simulink model "test"  (R2024b)
settings: Solver=VariableStepAuto  StartTime=0.0  StopTime=1  RelTol=1e-3
model workspace (MAT data in the model file):
  branch = 1
  resist = 1
values from neighbouring files (symbols this model uses):
  V = ww.ScopeData2.signals.values    [main.m]
libraries: spsCurrentMeasurementLib x1, spsPermanentMagnetSynchronousMachineLib x1, spsSeriesRLCBranchLib x1, spsUniversalBridgeLib x1, spsVoltageMeasurementLib x1, spsWindTurbineLib x1, sps_lib x1
settings Model: Creator=laity  LastModifiedBy=laity

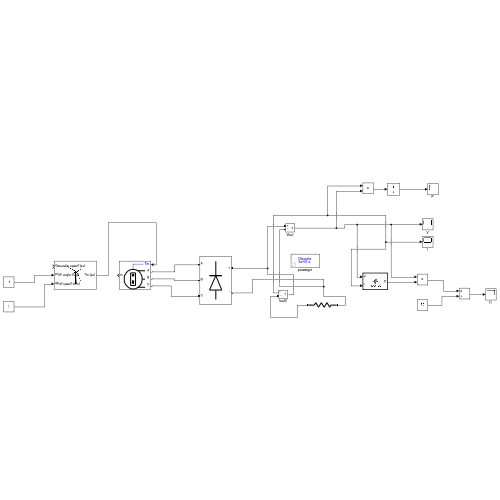
[thumbnail: Simulink's stored preview of the top-level diagram]
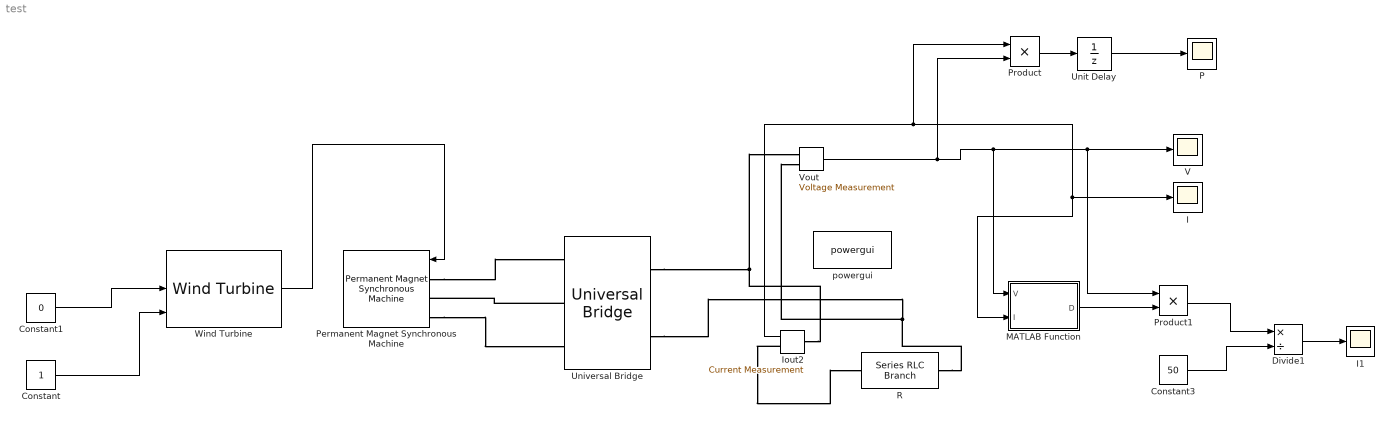
== system test ==
  Constant : Constant
  Constant1 : Constant  Value=0
  Constant3 : Constant  Value=50
  Divide1 : Product  Inputs=*/
  I : Scope
  I1 : Scope
  Iout2 : spsCurrentMeasurementLib/Current Measurement  PhasorSimulation=off  OutputType=Complex  PSBequivalent=0
  MATLAB Function : MATLAB Function  TreatAsAtomicUnit=on
  P : Scope
  Permanent Magnet Synchronous Machine : spsPermanentMagnetSynchronousMachineLib/Permanent Magnet Synchronous Machine  NbPhases=3  FluxDistribution=Sinusoidal  RotorType=Round  MechanicalLoad=Torque Tm  PresetModel=No  ShowDetailedParameters=on  MeasurementBus=off  Resistance=0.0485  Inductance=8.5e-3  dqInductances=[8.5e-3,8.5e-3]  La=0.000395  MachineConstant=Flux linkage established by magnets (V.s)  Flux=0.1194  VoltageCst=86.6271  TorqueCst=0.7164  Flat=120  Mechanical=[0.0027 0.0004924 4 0]  PolePairs=4  InitialConditions=[0,0, 0,0]  InitialConditions5ph=[0 0 0 0 0 0]  RefAngle=90 degrees behind phase A axis (modified Park)  IterativeDiscreteModel=Trapezoidal non iterative  TsBlock=-1  TsPowergui=0
  Product : Product
  Product1 : Product
  R : spsSeriesRLCBranchLib/Series RLC Branch  LConnTagsString=__new0  RConnTagsString=__new0  BranchType=R  Resistance=23.1298  Inductance=1e-3  SetiL0=off  InitialCurrent=0  Capacitance=1e-6  Setx0=off  InitialVoltage=0  Measurements=None
  Unit Delay : UnitDelay  SampleTime=-1  HasFrameUpgradeWarning=on
  Universal Bridge : spsUniversalBridgeLib/Universal Bridge  Arms=3  SnubberResistance=1e5  SnubberCapacitance=inf  Device=Diodes  Ron=1e-3  Lon=0  ForwardVoltages="[  0  0  ]"  ForwardVoltage=0  GTOparameters=[ 10e-6 , 20e-6 ]  IGBTparameters=[ 1e-6 , 2e-6 ]  Measurements=None  Measurements_2=None  converterType=Rectifier
  V : Scope
  Vout : spsVoltageMeasurementLib/Voltage Measurement  PhasorSimulation=off  OutputType=Complex  PSBequivalent=0
  Wind Turbine : spsWindTurbineLib/Wind Turbine  Pnom=1.5e6  Pelec_base=1.5e6/0.9  wind_base=12  P_wind_base=0.73  speed_nom=1.2  pitch_angle=0  c1_c6="[0.51763          116          0.4            5           21     0.006795]"  cp_nom=0.48  lambda_nom=8.1
  powergui : sps_lib/powergui  Priority=1  SimulationMode=Discrete  SampleTime=50e-6  frequency=60  Iterations=50  frequencyindice=0  Pbase=100e6  ErrMax=1e-4  UnitsV=kV  UnitsW=MW  buscounter=0  FunctionMessages=off  echomessages=off  EnableUseOfTLC=off  CurrentSourceSwitches=off  DisableSnubberDevices=off  DisableRonSwitches=off  DisableVfSwitches=off  DisplayEquations=off  AutomaticDiscreteSolvers=off  SolverType=Tustin/Backward Euler (TBE)  Interpol=off  ExternalGateDelay=off  methode=off  Ts=100  x0status=blocks  SPID=on  SwTol=0  HookPort=off  NonlinearTolerance=1e-4  nMaxIteration=100  ContinueOnMaxIteration=off  RestoreLinks=warning  ResistiveCurrentMeasurement=off  Frange=[0:2:500]  Ylog=off  Xlog=on  ShowGrid=off  save=off  variable=ZData  structure=0  ZoomFFT=off  StartTime=0.0  cycles=1  DisplayStyle=1  fundamental=60  FreqAxis=off  MaxFrequency=1000  frequencyindicesteady=1  RmsSteady=1  display=off
  wires:
  Vout/1 -> Product/2, MATLAB Function/1(V), Product1/1, V/1
  Iout2/1 -> Product/1, MATLAB Function/2(I), I/1
  Constant1/1 -> Wind Turbine/2
  Constant/1 -> Wind Turbine/3
  Wind Turbine/1 -> Permanent Magnet Synchronous Machine/1
  Unit Delay/1 -> P/1
  Product/1 -> Unit Delay/1
  MATLAB Function/1(D) -> Product1/2
  Product1/1 -> Divide1/1
  Constant3/1 -> Divide1/2
  Divide1/1 -> I1/1
  connections:
  Permanent Magnet Synchronous Machine/LConn1 -- Universal Bridge/LConn1
  Universal Bridge/LConn2 -- Permanent Magnet Synchronous Machine/LConn2
  Permanent Magnet Synchronous Machine/LConn3 -- Universal Bridge/LConn3
  Universal Bridge/RConn2 -- R/RConn1 -- Vout/LConn2
  Universal Bridge/RConn1 -- Iout2/LConn1 -- Vout/LConn1
  Iout2/RConn1 -- R/LConn1

== matlab function test/MATLAB Function ==
  data: V input; D output; I input
function D = mpo_po(V, I)
% persistent 状态
persistent Dk Pk
if isempty(Dk), Dk = 0.5; end
if isempty(Pk), Pk = 0;   end

P = V*I;
dP = P - Pk;

DeltaD = 0.005;                 % 步长
if abs(dP) < 0.002*max(P,1)     % 小功率变化死区（可调）
    DeltaD = 0.5*DeltaD;
end

if dP >= 0
    Dk = Dk + DeltaD;
else
    Dk = Dk - DeltaD;
end

Dk = min(max(Dk,0.02),0.98);    % 限幅
Pk = P;
D = Dk;
